simulink model "CompTorqueReg"  (R2019b)
settings: Solver=ode23s  StartTime=0.0  StopTime=25  RelTol=1e-3  AbsTol=1e-6
undefined symbols (not defined in the file): a0, a1, a2, a3, dq0, Kd_endEff, Kp_endEff, parameter, q0, x_endEff_D
libraries: simulink x1
settings Model: Creator=ariannagasparri  LastModifiedBy=ariannagasparri

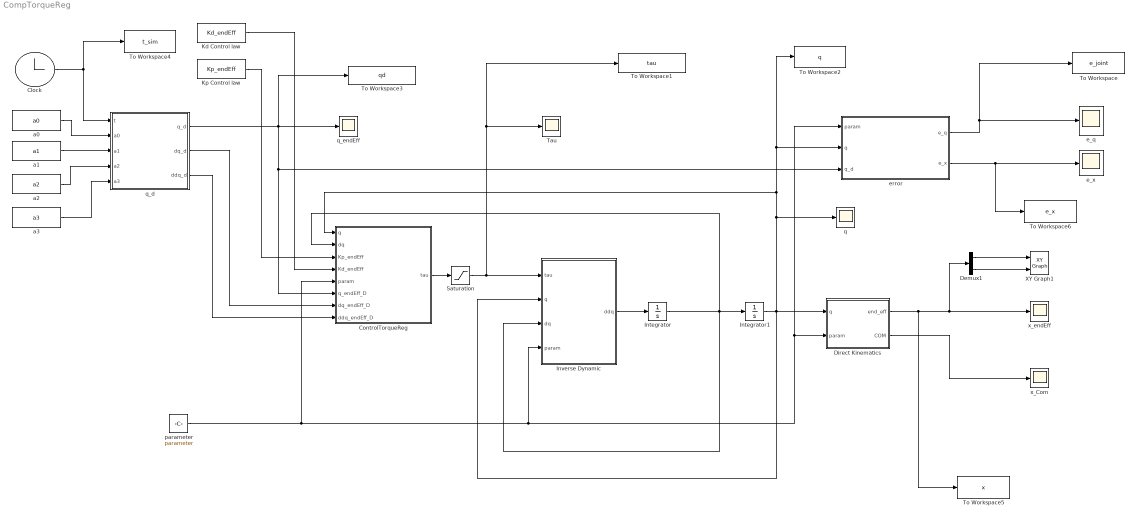
== system CompTorqueReg ==
  Clock : Clock
  ControlTorqueReg : MATLAB Function  TreatAsAtomicUnit=on
  Demux1 : Demux  Outputs=3
  "Direct Kinematics " : MATLAB Function  TreatAsAtomicUnit=on
  Integrator : Integrator  InitialCondition=dq0
  Integrator1 : Integrator  InitialCondition=q0
  "Inverse Dynamic " : MATLAB Function  TreatAsAtomicUnit=on
  Kd Control law : Constant  Value=Kd_endEff
  Kp Control law : Constant  Value=Kp_endEff
  Saturation : Saturate  UpperLimit=35000  LowerLimit=-35000
  Tau : Scope
  To Workspace : ToWorkspace  VariableName=e_joint  SaveFormat=Structure With Time  SampleTime=-1
  To Workspace1 : ToWorkspace  VariableName=tau  SaveFormat=Structure With Time  SampleTime=-1
  To Workspace2 : ToWorkspace  VariableName=q  SaveFormat=Structure With Time  SampleTime=-1
  To Workspace3 : ToWorkspace  VariableName=qd  SaveFormat=Structure With Time  SampleTime=-1
  To Workspace4 : ToWorkspace  VariableName=t_sim  SaveFormat=Structure With Time  SampleTime=-1
  To Workspace5 : ToWorkspace  VariableName=x  SaveFormat=Structure With Time  SampleTime=-1
  To Workspace6 : ToWorkspace  VariableName=e_x  SaveFormat=Structure With Time  SampleTime=-1
  XY Graph1 : simulink/Sinks/XY Graph  xmin=x_endEff_D(1)-2  xmax=x_endEff_D(1)+2  ymin=x_endEff_D(3)-2  ymax=x_endEff_D(3)+2  st=-1
  a0 : Constant  Value=a0
  a1 : Constant  Value=a1
  a2 : Constant  Value=a2
  a3 : Constant  Value=a3
  e_q : Scope
  e_x : Scope
  error : MATLAB Function  TreatAsAtomicUnit=on
  "parameter " : Constant  Value=parameter
  q : Scope
  q_d : MATLAB Function  TreatAsAtomicUnit=on
  q_endEff : Scope
  x_Com : Scope
  x_endEff : Scope
  wires:
  a0/1 -> q_d/2(a0)
  "parameter "/1 -> ControlTorqueReg/5(param), error/1(param), "Direct Kinematics "/2(param), "Inverse Dynamic "/4(param)
  Integrator/1 -> ControlTorqueReg/2(dq), "Inverse Dynamic "/3(dq), Integrator1/1
  "Inverse Dynamic "/1(ddq) -> Integrator/1
  Integrator1/1 -> "Direct Kinematics "/1(q), To Workspace2/1, error/2(q), ControlTorqueReg/1(q), q/1, "Inverse Dynamic "/2(q)
  q_d/3(ddq_d) -> ControlTorqueReg/8(ddq_endEff_D)
  Clock/1 -> q_d/1(t), To Workspace4/1
  Demux1/3 -> XY Graph1/2
  a2/1 -> q_d/4(a2)
  Demux1/1 -> XY Graph1/1
  error/1(e_q) -> To Workspace/1, e_q/1
  error/2(e_x) -> To Workspace6/1, e_x/1
  q_d/2(dq_d) -> ControlTorqueReg/7(dq_endEff_D)
  a1/1 -> q_d/3(a1)
  Saturation/1 -> "Inverse Dynamic "/1(tau), To Workspace1/1, Tau/1
  q_d/1(q_d) -> ControlTorqueReg/6(q_endEff_D), error/3(q_d), To Workspace3/1, q_endEff/1
  "Direct Kinematics "/1(end_eff) -> To Workspace5/1, Demux1/1, x_endEff/1
  Kp Control law/1 -> ControlTorqueReg/3(Kp_endEff)
  ControlTorqueReg/1(tau) -> Saturation/1
  a3/1 -> q_d/5(a3)
  "Direct Kinematics "/2(COM) -> x_Com/1
  Kd Control law/1 -> ControlTorqueReg/4(Kd_endEff)

== matlab function CompTorqueReg/Direct Kinematics  ==
  data: q input; end_eff output; param input; COM output
function [end_eff, COM] = DirectK(q,param)


    [Pcom, Etip,T00,T01,T12,T23,T34,T45,T56] =  forwardKinematics(param, q);
    
    
    end_eff = Etip(1:3,4);
    COM = Pcom;
    
end

== matlab function CompTorqueReg/Inverse Dynamic  ==
  data: tau input; q input; dq input; ddq output; param input
function ddq = inverseDynamic(tau,q,dq,param)

    B = B_fun(param, q);
    C = C_fun(param, q, dq);
    G = G_fun(param, q);

    ddq = B\(tau - G - C*dq);

end

== matlab function CompTorqueReg/ControlTorqueReg ==
  data: q input; dq input; Kp_endEff input; Kd_endEff input; tau output; param input; q_endEff_D input; dq_endEff_D input; ddq_endEff_D input
function tau  = x_now(q, dq, Kp_endEff, Kd_endEff, param, q_endEff_D, dq_endEff_D, ddq_endEff_D)

%     g0 = 9.81;
    Y = Y_fun(param, q, dq, ddq_endEff_D);
    Pi = [param(6,2); 1];
    
%     Kp_endEff = K_endEff(1);
%     Kd_endEff = K_endEff(2);

    %% controllo Diretto
    
    e_endEff = q_endEff_D - q;
    de_endEff = dq_endEff_D - dq;
    
%     tau = Kp_endEff*e_endEff + Kd_endEff*de_endEff + G + C*dq + B*ddq_endEff_D;
    tau = Y*Pi + Kp_endEff*e_endEff + Kd_endEff*de_endEff;
    
end

== matlab function CompTorqueReg/error ==
  data: param input; q input; e_q output; q_d input; e_x output
function [e_q, e_x]  = error(param, q, q_d)
    

%     [~, Etip,~,~,~,~,~,~,~] =  forwardKinematics(param, q*pi/180);
%     [~, Etip_d,~,~,~,~,~,~,~] =  forwardKinematics(param, q_d*pi/180);  

    [~, Etip,~,~,~,~,~,~,~] =  forwardKinematics(param, q);
    [~, Etip_d,~,~,~,~,~,~,~] =  forwardKinematics(param, q_d);  

    e_x = Etip_d(1:3,4) - Etip(1:3,4);

    e_q = q_d - q;
    
end

== matlab function CompTorqueReg/q_d ==
  data: t input; q_d output; dq_d output; ddq_d output; a0 input; a1 input; a2 input; a3 input
function [q_d,dq_d,ddq_d] = desiderable_q(t, a0,a1,a2,a3)

    [q_d, dq_d, ddq_d] = vettoreq(a0,a1,a2,a3,t);
    
end
